simulink model "MSDR_v1"  (R2018a)
settings: Solver=ode23tb  StartTime=0.0  StopTime=50000  RelTol=1e-3
values from neighbouring files (symbols this model uses):
  a_f = -3.22E-5    (= -3.22e-05)    [MSDR_parameters.m]
  a_g = +2.35E-5    (= 2.35e-05)    [MSDR_parameters.m]
  beta = [0.000223, 0.001457, 0.001307, 0.002628, 0.000766, 0.000280]    [MSDR_parameters.m]
  beta_t = sum(beta)    [MSDR_parameters.m]
  Cp_s_shx = 1549.12e-6    (= 0.00154912)    [MSDR_parameters.m]
  Cst = 10    [MSDR_parameters.m]
  dLb = 0    [MSDR_parameters.m]
  dLs = 0    [MSDR_parameters.m]
  dLsc = 0    [MSDR_parameters.m]
  gamma_I = 5.1135e-2    (= 0.051135)    [MSDR_parameters.m]
  gamma_Xe = 1.1628e-2    (= 0.011628)    [MSDR_parameters.m]
  hA_fg = [h_fg*A_fg/2, h_fg*A_fg/2]    [MSDR_parameters.m]
  hA_p_phx1 = h_p_phx*A_p_phx    [MSDR_parameters.m]
  hA_p_phx2 = h_p_phx*A_p_phx    [MSDR_parameters.m]
  hA_p_phx3 = h_p_phx*A_p_phx    [MSDR_parameters.m]
  hA_p_phx4 = h_p_phx*A_p_phx    [MSDR_parameters.m]
  hA_p_phx5 = h_p_phx*A_p_phx    [MSDR_parameters.m]
  hA_p_phx6 = h_p_phx*A_p_phx    [MSDR_parameters.m]
  hA_p_shx1 = h_p_shx*A_p_shx    [MSDR_parameters.m]
  hA_p_shx2 = h_p_shx*A_p_shx    [MSDR_parameters.m]
  hA_p_shx3 = h_p_shx*A_p_shx    [MSDR_parameters.m]
  hA_p_shx4 = h_p_shx*A_p_shx    [MSDR_parameters.m]
  hA_p_shx5 = h_p_shx*A_p_shx    [MSDR_parameters.m]
  hA_p_shx6 = h_p_shx*A_p_shx    [MSDR_parameters.m]
  hA_s_phx1 = h_s_phx*A_s_phx    [MSDR_parameters.m]
  hA_s_phx2 = h_s_phx*A_s_phx    [MSDR_parameters.m]
  hA_s_phx3 = h_s_phx*A_s_phx    [MSDR_parameters.m]
  hA_s_phx4 = h_s_phx*A_s_phx    [MSDR_parameters.m]
  hA_s_phx5 = h_s_phx*A_s_phx    [MSDR_parameters.m]
  hA_s_phx6 = h_s_phx*A_s_phx    [MSDR_parameters.m]
  hA_s_shx1 = h_s_shx*A_s_shx    [MSDR_parameters.m]
  hA_s_shx2 = h_s_shx*A_s_shx    [MSDR_parameters.m]
  hA_s_shx3 = h_s_shx*A_s_shx    [MSDR_parameters.m]
  hA_s_shx4 = h_s_shx*A_s_shx    [MSDR_parameters.m]
  hA_s_shx5 = h_s_shx*A_s_shx    [MSDR_parameters.m]
  hA_s_shx6 = h_s_shx*A_s_shx    [MSDR_parameters.m]
  I_0 = gamma_I*Sig_f_msdr*phi_0/lam_I    (= 4.38204721773e+16)    [MSDR_parameters.m]
  Ifa = [0.25, 0.25]    [MSDR_parameters.m]
  Ifb = [0.25, 0.25]    [MSDR_parameters.m]
  Ig = [0.5, 0.5]    [MSDR_parameters.m]
  J = 1e-6    (= 1e-06)    [MSDR_parameters.m]
  ka = [0.235, 0.235]    [MSDR_parameters.m]
  kb = [0.235, 0.235]    [MSDR_parameters.m]
  kc = 5    [MSDR_parameters.m]
  kga = [0.015, 0.015]    [MSDR_parameters.m]
  kgb = [0.015, 0.015]    [MSDR_parameters.m]
  L = 8.5344    [MSDR_parameters.m]
  Lam = 2.400E-04    (= 0.00024)    [MSDR_parameters.m]
  lam = [0.0124, 0.0305, 0.111, 0.301, 1.14, 3.01]    [MSDR_parameters.m]
  lam_bubl = 2.0e-2    (= 0.02)    [MSDR_parameters.m]
  lam_I = 2.875e-5    (= 2.875e-05)    [MSDR_parameters.m]
  lam_Xe = 2.0916e-5    (= 2.0916e-05)    [MSDR_parameters.m]
  m_3m = W_3*2    (= 8618.207327)    [MSDR_parameters.m]
  m_fm = W_f*2    (= 9978.96)    [MSDR_parameters.m]
  m_sb = 1717    [MSDR_parameters.m]
  mb_cpb = 2.689619410657651e+00    (= 2.68961941066)    [MSDR_parameters.m]
  mcp_fa = mfa*Cp_f    [MSDR_parameters.m]
  mcp_fb = mfb*Cp_f    [MSDR_parameters.m]
  mcp_g = mg*Cp_g    [MSDR_parameters.m]
  mcp_p_phx1 = Cp_p_phx*mp_phx1    [MSDR_parameters.m]
  mcp_p_phx2 = Cp_p_phx*mp_phx2    [MSDR_parameters.m]
  mcp_p_phx3 = Cp_p_phx*mp_phx3    [MSDR_parameters.m]
  mcp_p_phx4 = Cp_p_phx*mp_phx4    [MSDR_parameters.m]
  mcp_p_phx5 = Cp_p_phx*mp_phx5    [MSDR_parameters.m]
  mcp_p_phx6 = Cp_p_phx*mp_phx6    [MSDR_parameters.m]
  mcp_p_shx1 = Cp_p_shx*mp_shx1    [MSDR_parameters.m]
  mcp_p_shx2 = Cp_p_shx*mp_shx2    [MSDR_parameters.m]
  mcp_p_shx3 = Cp_p_shx*mp_shx3    [MSDR_parameters.m]
  mcp_p_shx4 = Cp_p_shx*mp_shx4    [MSDR_parameters.m]
  mcp_p_shx5 = Cp_p_shx*mp_shx5    [MSDR_parameters.m]
  mcp_p_shx6 = Cp_p_shx*mp_shx6    [MSDR_parameters.m]
  mcp_s_phx1 = Cp_s_phx*ms_phx1    [MSDR_parameters.m]
  mcp_s_phx2 = Cp_s_phx*ms_phx2    [MSDR_parameters.m]
  mcp_s_phx3 = Cp_s_phx*ms_phx3    [MSDR_parameters.m]
  mcp_s_phx4 = Cp_s_phx*ms_phx4    [MSDR_parameters.m]
  mcp_s_phx5 = Cp_s_phx*ms_phx5    [MSDR_parameters.m]
  mcp_s_phx6 = Cp_s_phx*ms_phx6    [MSDR_parameters.m]
  mcp_s_shx1 = Cp_s_shx*ms_shx1    [MSDR_parameters.m]
  mcp_s_shx2 = Cp_s_shx*ms_shx1    [MSDR_parameters.m]
  mcp_s_shx3 = Cp_s_shx*ms_shx1    [MSDR_parameters.m]
  mcp_s_shx4 = Cp_s_shx*ms_shx1    [MSDR_parameters.m]
  mcp_s_shx5 = Cp_s_shx*ms_shx1    [MSDR_parameters.m]
  mcp_s_shx6 = Cp_s_shx*ms_shx1    [MSDR_parameters.m]
  mcp_t_phx1 = Cp_t_phx*mt_phx1    [MSDR_parameters.m]
  mcp_t_phx2 = Cp_t_phx*mt_phx2    [MSDR_parameters.m]
  mcp_t_phx3 = Cp_t_phx*mt_phx3    [MSDR_parameters.m]
  mcp_t_phx4 = Cp_t_phx*mt_phx4    [MSDR_parameters.m]
  mcp_t_phx5 = Cp_t_phx*mt_phx5    [MSDR_parameters.m]
  mcp_t_phx6 = Cp_t_phx*mt_phx6    [MSDR_parameters.m]
  mcp_t_shx1 = Cp_t_phx*mt_shx1    [MSDR_parameters.m]
  mcp_t_shx2 = Cp_t_phx*mt_shx2    [MSDR_parameters.m]
  mcp_t_shx3 = Cp_t_phx*mt_shx3    [MSDR_parameters.m]
  mcp_t_shx4 = Cp_t_phx*mt_shx4    [MSDR_parameters.m]
  mcp_t_shx5 = Cp_t_phx*mt_shx5    [MSDR_parameters.m]
  mcp_t_shx6 = Cp_t_phx*mt_shx6    [MSDR_parameters.m]
  mfa = [mass_fn, mass_fn]    [MSDR_parameters.m]
  mfb = [mass_fn, mass_fn]    [MSDR_parameters.m]
  mp_phx1 = [494.7, 494.7, 494.7, 494.7]    [MSDR_parameters.m]
  mp_phx2 = [494.7, 494.7, 494.7, 494.7]    [MSDR_parameters.m]
  mp_phx3 = [494.7, 494.7, 494.7, 494.7]    [MSDR_parameters.m]
  mp_phx4 = [494.7, 494.7, 494.7, 494.7]    [MSDR_parameters.m]
  mp_phx5 = [494.7, 494.7, 494.7, 494.7]    [MSDR_parameters.m]
  mp_phx6 = [494.7, 494.7, 494.7, 494.7]    [MSDR_parameters.m]
  mp_phxm = (Wp_phx1 + Wp_phx2)*1    (= 1663.16)    [MSDR_parameters.m]
  mp_shx1 = [429.3, 429.3, 429.3, 429.3]    [MSDR_parameters.m]
  mp_shx2 = [429.3, 429.3, 429.3, 429.3]    [MSDR_parameters.m]
  mp_shx3 = [429.3, 429.3, 429.3, 429.3]    [MSDR_parameters.m]
  mp_shx4 = [429.3, 429.3, 429.3, 429.3]    [MSDR_parameters.m]
  mp_shx5 = [429.3, 429.3, 429.3, 429.3]    [MSDR_parameters.m]
  mp_shx6 = [429.3, 429.3, 429.3, 429.3]    [MSDR_parameters.m]
  mp_shxm = (Wp_shx1 + Wp_shx2)*1    (= 932.38)    [MSDR_parameters.m]
  ms_phx1 = [1152.5, 1152.5, 1152.5, 1152.5]    [MSDR_parameters.m]
  ms_phx2 = [1152.5, 1152.5, 1152.5, 1152.5]    [MSDR_parameters.m]
  ms_phx3 = [1152.5, 1152.5, 1152.5, 1152.5]    [MSDR_parameters.m]
  ms_phx4 = [1152.5, 1152.5, 1152.5, 1152.5]    [MSDR_parameters.m]
  ms_phx5 = [1152.5, 1152.5, 1152.5, 1152.5]    [MSDR_parameters.m]
  ms_phx6 = [1152.5, 1152.5, 1152.5, 1152.5]    [MSDR_parameters.m]
  ms_phxm = (Ws_phx1 + Ws_phx2)*1    (= 932.38)    [MSDR_parameters.m]
  ms_shx1 = [1861.5, 1861.5, 1861.5, 1861.5]    [MSDR_parameters.m]
  ms_shx2 = [1861.5, 1861.5, 1861.5, 1861.5]    [MSDR_parameters.m]
  ... (+104 more)
undefined symbols (not defined in the file or in its folder): Ak2, As, C0, Cpp, Cps, Cpsc, Cpw, Dit, Dot, hA_p_thx1, hA_p_thx2, hA_p_thx3, hA_s_thx1, hA_s_thx2, hA_s_thx3, hc0, hfg, hfw0, HFW1, hfw10, HFW2, hpw, Hr, hr0, hwb, hws, hwsc, K3, KBHP, KBLP, Lsc, mcp_p_thx1, mcp_p_thx2, mcp_p_thx3, mcp_s_thx1, mcp_s_thx2, mcp_s_thx3, mcp_t_thx1, mcp_t_thx2, mcp_t_thx3, mp_thx1, mp_thx2, mp_thx3, ms_thx1, ms_thx2, ms_thx3, Mstm, nuf, Pp2, Pp3, Pp4, Pp5
libraries: simulink x20, aerolibconvert2 x2
(part 3 of 7)

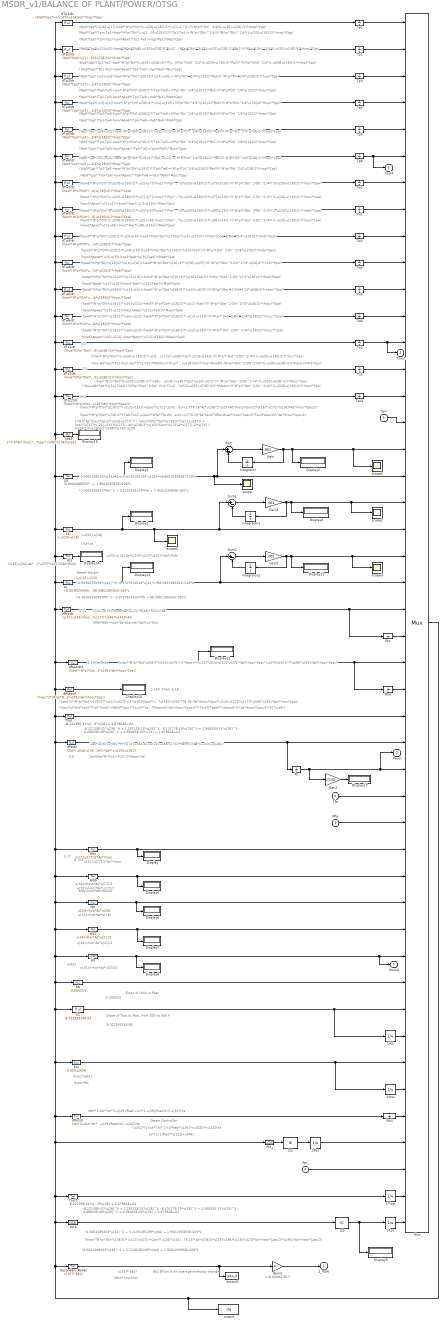
== system MSDR_v1/BALANCE OF PLANT/POWER/OTSG ==
  note: 1/(0.5*As*rhosc*Cpsc*(u[15]-u[27])) * ( hwsc*(N*pi*Dot*u[18]/2)*(u[11]-u[27]) + Cpsc*(u[31]*u[15]-u[32]*u[27]) - As*u[18]/2*(u[40]*Cpsc*(u[15]-2*u[27])-1)*u[23] ) - 0.5*As*rhosc*Cpsc*u[38]*u[18]*u[25]
  note: (u[33]-u[34]-As*u[20]*u[37]*u[25])/(As*rhob)
  note: 3.31 Ke Zhao
  note: rhosc*u[43]
  note: rhosc/Psc
  note: (Ws*(1-Cst*(kc*(1-u[29]/Pset)+kc*(1-u[29]/Pset)/ti))-u[42])/ts
  note: u[42]
  note: (0.0001589253*u[44]^2 + 0.1130185109*u[44] + 1.9561035858)/100*L
  note: (hwsc*2*(N*pi*Dot*u[18]/2)*(u[11]-u[27])+2*u[35]*Cpsc*(u[15]-u[27])-u[25]*As*u[18]*u[40]*Cpsc*(u[15]-2*u[27])+(As*u[18]*u[25]/778.16)-As*rhosc*Cpsc*(u[15]-u[27])*u[17])*u[46]*u[39]/(As*rhosc*Cpsc)
  note: u[31]-u[17]/2*As*rhosc
  note: ((hws*(N*pi*Dot*(L-u[20]-u[18])/2)*(u[8]-u[14]))-u[30]*Cps*(u[14]-u[27]))/(((N*pi*(Dot^2-Dit^2)/4*((L-u[20]-u[18])/2))*rhos)*Cps)
  note: ((hws*(N*pi*Dot*(L-u[20]-u[18])/2)*(u[7]-u[13]))-u[36]*Cps*(u[13]-u[14]))/(((N*pi*(Dot^2-Dit^2)/4*((L-u[20]-u[18])/2))*rhos)*Cps)
  note: (0.0001589253*u[44]^2 + 0.1130185109*u[44] + 1.9561035858)/100*L
  note: 882 BTU/s is an average enthalpy change
  note: u[33]*(882)
  note: Wfw*(hms-hfw)
  note: (-0.0036059099*Pth^2 - 0.3727634534*Pth + 88.5961185354)/100*L
  note: (-0.0036059099*u[44]^2 - 0.3727634534*u[44] + 88.5961185354)/100*L
  note: L-u[22]-u[18]
  note: L-Ls-Lsc
  note: (0.0001589253*Pth^2 + 0.1130185109*Pth + 1.9561035858)/100*L
  note: (0.0001589253*u[44]^2 + 0.1130185109*u[44] + 1.9561035858)/100*L
  note: 5.6
  note: u[31]+rhos*As*u[21]/2
  note: -8.22139E-31*u[26]^6 + 1.29715E-24*u[26]^5 - 8.10177E-19*u[26]^4 + 2.56855E-13*u[26]^3 - 4.48833E-08*u[26]^2 + 4.96063E-03*u[26] + 2.67964E+02
  note: Wfw-rhosc*As*dLscdt
  note: Steam Height
  note: Steam Controller
  note: (u[31]*(1-Cst*((kc*(1-(1/Pset)*u[29])+u[43])))-u[42])/ts
  note: L-u[18]-u[20]
  note: 8.02299324E-04
  note: -0.000053
  note: (u[31]-u[33]-rhosc*As*u[17])*u[46]*u[41]/(As)
  note: u[34]-rhos*As*u[21]/2
  note: -8.22139E-31*u[26]^6 + 1.29715E-24*u[26]^5 - 8.10177E-19*u[26]^4 + 2.56855E-13*u[26]^3 - 4.48833E-08*u[26]^2 + 4.96063E-03*u[26] + 2.67964E+02
  note: (hwsc*(N*pi*Dot*u[18]/2)*(u[11]-u[27])+Cpsc*(u[28]*u[15]-u[29]*u[27])+(1/778.16)*As*u[18]/2*u[25]-u[38]*u[18]*u[23]*As*rhosc*Cpsc/2)*u[38]/(As*rhosc*Cpsc/2)
  note: u[32]-rhosc*As*u[17]/2
  note: 5.17
  note: (Wfw-Wdb-rhosc*As*dLsc/dt)/(As*Lsc*Ksc)
  note: 5.13
  note: u[33]-rhob*As*u[19]
  note: 5.11
  note: 5.5
  note: 5.4
  note: ((Qs2-Wb*Cps*(u[14]-Tsat)-(((N*pi*(Dot^2-Dit^2)/4*((L-u[20]-u[18])/2))*rhos)*dHsdPs-(N*pi*(Dot^2-Dit^2)/4*((L-u[20]-u[18])/2)))*Pdots))/(((N*pi*(Dot^2-Dit^2)/4*((L-u[20]-u[18])/2))*rhos)*Cps)
  note: (Qs1-Ws*Cps*(Ts1-Ts2)-Cps*(Ts1-Ts2)*Mdots1-((N*pi*(Dot^2-Dit^2)/4*((L-u[20]-u[18])/2))*rhos)*dHsdPs-(N*pi*(Dot^2-Dit^2)/4*((L-u[20]-u[18])/2))*Pdots)/(Ms1*Cps)
  note: (hpw4*(N*pi*Dit*u[20]/2)*(u[4]-u[10])-hws4*(N*pi*Dot*u[20]/2)*(u[10]-Tsat))/(((N*pi*(Dot^2-Dit^2)/4*u[20]/2)*rhob)*Cpw)
  note: (hpw3*(N*pi*Dit*u[20]/2)*(u[3]-u[9])-hws3*(N*pi*Dot*u[20]/2)*(u[9]-Tsat))/(((N*pi*(Dot^2-Dit^2)/4*u[20]/2)*rhob)*Cpw)
  note: (hpw2*(N*pi*Dit*(L-u[20]-u[18])/2)*(u[2]-u[8])-hws2*(N*pi*Dot*(L-u[20]-u[18])/2)*(u[8]-u[14]))/(((N*pi*(Dot^2-Dit^2)/4*((L-u[20]-u[18])/2))*rhos)*Cpw)
  note: (hpw1*(N*pi*Dit*(L-u[20]-u[18])/2)*(u[1]-u[7])-hws1*(N*pi*Dot*(L-u[20]-u[18])/2)*(u[7]-u[13]))/(((N*pi*(Dot^2-Dit^2)/4*((L-u[20]-u[18])/2))*rhos)*Cpw)
  note: (Wp0*Cpp*(Tp3-Tp4)-hpw*(N*pi*Dit*u[20]/2)*(Tp4-Tw4)+(N*pi*Dit^2/4*u[20]/2)*Pp4)/(((N*pi*Dit^2/4*u[20]/2)*rhop)*Cpp)
  note: (Wp0*Cpp*(Tp2-Tp3)-hpw*(N*pi*Dit*u[20]/2)*(Tp3-Tw3)+(N*pi*Dit^2/4*u[20]/2)*Pp3)/(((N*pi*Dit^2/4*u[20]/2)*rhop)*Cpp)
  note: (Wp0*Cpp*(Tp1-Tp2)-hpw*(N*pi*Dit*(L-u[20]-u[18])/2)*(Tp2-Tw2)+(N*pi*(Dit)^2/4*(L-u[20]-u[18])/2)*Pp2)/(((N*pi*(Dit)^2/4*(L-u[20]-u[18])/2)*rhop)*Cpp)
  note: (Wp0*Cpp*(Tpin-Tp1)-hpw*(N*pi*Dit*(L-u[20]-u[18])/2)*(Tp1-Tw1)+(N*pi*(Dit)^2/4)/(((N*pi*(Dit)^2/4*(L-u[20]-u[18])/2)*rhop)*Cpp)
  note: (Wp0*Cpp*(Tp4-Tp5)-hpw*(N*pi*Dit*u[18]/2)*(Tp5-Tw5)+(N*pi*Dit^2/4*u[18]/2)*Pp5)/(((N*pi*Dit^2/4*u[18]/2)*rhop)*Cpp)
  note: (Wp0*Cpp*(Tp5-Tp6)-hpw*(N*pi*Dit*u[18]/2)*(Tp6-Tw6)+(N*pi*Dit^2/4*u[18]/2)*Pp6)/(((N*pi*Dit^2/4*u[18]/2)*rhop)*Cpp)
  note: (hpw6*(N*pi*Dit*u[18]/2)*(u[6]-u[12])-hws6*(N*pi*Dot*u[18]/2)*(u[12]-u[18]))/(((N*pi*(Dot^2-Dit^2)/4*u[18]/2)*rhosc)*Cpw)
  note: (hpw5*(N*pi*Dit*u[18]/2)*(u[5]-u[11])-hws5*(N*pi*Dot*u[18]/2)*(u[11]-Tsat))/(((N*pi*(Dot^2-Dit^2)/4*u[18]/2)*rhosc)*Cpw)
  note: (hwsc*(N*pi*Dot*u[18]/2)*(Tw6-Tsc2)+Cpsc*(Wfw*Tfw-Wsc*Tsc2)+1/778.16*As*Lsc/2*dPsc/dt-As*rhosc*Cpsc/2*Tsc2*dLsc/dt)/(As*rhosc*Cpsc/2)
  note: (Wp0*Cpp*(u[16]-u[1])-hpw*(N*pi*Dit*(L-u[20]-u[18])/2)*(u[1]-u[7]))/(((N*pi*(Dit)^2/4*(L-u[20]-u[18])/2)*rhop)*Cpp)
  note: (Wp0*Cpp*(u[1]-u[2])-hpw*(N*pi*Dit*(L-u[20]-u[18])/2)*(u[2]-u[8])+(N*pi*(Dit)^2/4*(L-u[20]-u[18])/2)*Pp2)/(((N*pi*(Dit)^2/4*(L-u[20]-u[18])/2)*rhop)*Cpp)
  note: (Wp0*Cpp*(u[2]-u[3])-hpw*(N*pi*Dit*u[20]/2)*(u[3]-u[9])+(N*pi*Dit^2/4*u[20]/2)*Pp3)/(((N*pi*Dit^2/4*u[20]/2)*rhop)*Cpp)
  note: (Wp0*Cpp*(u[3]-u[4])-hpw*(N*pi*Dit*u[20]/2)*(u[4]-u[10])+(N*pi*Dit^2/4*u[20]/2)*Pp4)/(((N*pi*Dit^2/4*u[20]/2)*rhop)*Cpp)
  note: (Wp0*Cpp*(u[5]-u[6])-hpw*(N*pi*Dit*u[18]/2)*(u[6]-u[12])+(N*pi*Dit^2/4*u[18]/2)*Pp6)/(((N*pi*Dit^2/4*u[18]/2)*rhop)*Cpp)
  note: (Wp0*Cpp*(u[4]-u[5])-hpw*(N*pi*Dit*u[18]/2)*(u[5]-u[11])+(N*pi*Dit^2/4*u[18]/2)*Pp5)/(((N*pi*Dit^2/4*u[18]/2)*rhop)*Cpp)
  note: (hpw1*(N*pi*Dit*(L-u[20]-u[18])/2)*(u[1]-u[7])-hws1*(N*pi*Dot*(L-u[20]-u[18])/2)*(u[7]-u[13]))/(((N*pi*(Dot^2-Dit^2)/4*((L-u[20]-u[18])/2))*rhos)*Cpw)
  note: (hpw2*(N*pi*Dit*(L-u[20]-u[18])/2)*(u[2]-u[8])-hws2*(N*pi*Dot*(L-u[20]-u[18])/2)*(u[8]-u[14]))/(((N*pi*(Dot^2-Dit^2)/4*((L-u[20]-u[18])/2))*rhos)*Cpw)
  note: (hpw3*(N*pi*Dit*u[20]/2)*(u[3]-u[9])-hws3*(N*pi*Dot*u[20]/2)*(u[9]-u[27]))/(((N*pi*(Dot^2-Dit^2)/4*u[20]/2)*rhob)*Cpw)
  note: (hpw4*(N*pi*Dit*u[20]/2)*(u[4]-u[10])-hws4*(N*pi*Dot*u[20]/2)*(u[10]-u[27]))/(((N*pi*(Dot^2-Dit^2)/4*u[20]/2)*rhob)*Cpw)
  note: (hpw5*(N*pi*Dit*u[18]/2)*(u[5]-u[11])-hws5*(N*pi*Dot*u[18]/2)*(u[11]-u[27]))/(((N*pi*(Dot^2-Dit^2)/4*u[18]/2)*rhosc)*Cpw)
  note: (hpw6*(N*pi*Dit*u[18]/2)*(u[6]-u[12])-hws6*(N*pi*Dot*u[18]/2)*(u[12]-u[15]))/(((N*pi*(Dot^2-Dit^2)/4*u[18]/2)*rhosc)*Cpw)
  note: (hwsc*pi*Dot*Lsc0*(Tw5-Tsat0)+Wfw0*Cpsc*(Tsc20-Tsat0)-((As*Lsc0/2)*(Ksc*Cpsc*(Tsc20-2*Tsat0)-1/778)*Pdotsc0)-(As*rhosc*Cpsc/2*((Tsc20-Tsat0)*Ldotsc0)))/(As*rhosc*Cpsc/2*(K1*Lsc0))
  note: p.152
  note: p.153, Chen, 5.18
  note: Zss*Mss*R*(Ts1+Ts2)/(2*Mstm*Vs)
  note: (Zss*(u[34]-u[36])*R*(u[13]+458.67+u[14]+458.67)/(2*Mstm))/(As*(L-u[20]-u[18]))
  note: Slope of Tsat vs Psat, from 500 to 600 F
  note: Slope of rhob vs Psat
  note: (Wp0*Cpp*(Tpin-Tp1)-hpw*Apws*(Tp1-Tw1)+Vps*Pp1)/(Mps*Cpp)
  note: (Wp0*Cpp*(Tp1-Tp2)-hpw*Apws*(Tp2-Tw2)+Vps*Pp2)/(Mps*Cpp)
  note: (Wp0*Cpp*(Tp2-Tp3)-hpw*Apwb*(Tp3-Tw3)+Vpb*Pp3)/(Mpb*Cpp)
  note: (Wp0*Cpp*(Tp3-Tp4)-hpw*Apwb*(Tp4-Tw4)+Vpb*Pp4)/(Mpb*Cpp)
  note: (Wp0*Cpp*(Tp4-Tp5)-hpw*Apwsc*(Tp5-Tw5)+Vpsc*Pp5)/(Mpsc*Cpp)
  note: (Wp0*Cpp*(Tp5-Tp6)-hpw*Apwsc*(Tp6-Tw6)+Vpsc*Pp6)/(Mpsc*Cpp)
  note: (hpw1*Apws*(u[1]-u[7])-hws1*Aws*(u[7]-u[13]))/(Mws*Cpw)
  note: (hpw2*Apws*(u[2]-u[8])-hws2*Aws*(u[8]-u[14]))/(Mws*Cpw)
  note: (hpw3*Apwb*(u[3]-u[9])-hws3*Awb*(u[9]-Tsat))/(Mwb*Cpw)
  note: (hpw4*Apwb*(u[4]-u[10])-hws4*Awb*(u[10]-Tsat))/(Mwb*Cpw)
  note: (hpw5*Apwsc*(u[5]-u[11])-hwsc*Awsc*(u[11]-Tsat))/(Mwsc*Cpw)
  note: (hpw6*Apwsc*(u[6]-u[12])-hwsc*Awsc*(u[12]-u[18]))/(Mwsc*Cpw)
  note: kc*(1-(1/Pset)*u[22])+u[46]
  note: (hwsc*(N*pi*Dot*u[18]/2)*(u[12]-u[15])+Cpsc*(u[31]*u[30]-u[32]*u[15])+1/778.16*As*u[18]/2*u[23]-As*rhosc*Cpsc/2*u[15]*u[17])/(u[18]*As*rhosc*Cpsc/2)
  note: (hwsc*(N*pi*Dot*u[18])*(u[11]-u[27])+2*Cpsc*(u[32]*u[15]-u[33]*u[27])-(As*rhosc*Cpsc*(u[27]*u[17])))*u[46]*u[39]/(As*rhosc*Cpsc)
  Wfw : Inport
  Tfw : Inport  Port=2
  Tpin : Inport  Port=3
  Pth_ : Inport  Port=4
  1/K1 : Math  Operator=reciprocal  SaturateOnIntegerOverflow=on
  1/Ksc : Math  Operator=reciprocal  SaturateOnIntegerOverflow=on
  1/Lsc : Math  Operator=reciprocal  SaturateOnIntegerOverflow=on
  1/Psc : Math  Operator=reciprocal  SaturateOnIntegerOverflow=on
  1/Tsat : Math  Operator=reciprocal  SaturateOnIntegerOverflow=on
  Display{,1..16} (17 alike) : Display
  Gain : Gain  Gain=.001
  Gain1 : Gain  Gain=.001
  Gain2 : Gain  Gain=.001
  Gain3 : Gain  Gain=1./0.000947817
  Gan2 : Gain  Gain=1/144
  IC2 : InitialCondition  Value=Psc
  IC9 : InitialCondition  Value=Lsc
  Integrator : Integrator  InitialCondition=dLsc
  Integrator1 : Integrator  InitialCondition=dLb
  Integrator2 : Integrator  InitialCondition=dLs
  K1 : Fcn  Expr=8.02299324E-04
  Kb : Fcn  Expr=-0.000053
  Ksc : Fcn  Expr=0.00042636
  Lb : Fcn  Expr=L-u[22]-u[18]
  Lb1 : Fcn  Expr=(u[33]-u[34]-As*u[20]*u[37]*u[25])/(As*rhob)
  Ls : Fcn  Expr=(-0.0036059099*u[44]^2 - 0.3727634534*u[44] + 88.5961185354)/100*L
  Lsc : Fcn  Expr=(0.0001589253*u[44]^2 + 0.1130185109*u[44] + 1.9561035858)/100*L
  Lsc1 : Fcn  Expr=u[18]
  Lsc2 : Fcn  Expr="1/(0.5*As*rhosc*Cpsc*(u[15]-u[27])) * (  hwsc*(N*pi*Dot*u[18]/2)*(u[11]-u[27])  +  Cpsc*(u[31]*u[15]-u[32]*u[27])  -  As*u[18]/2*(u[40]*Cpsc*(u[15]-2*u[27])-1)*u[23]  )  -  0.5*As*rhosc*Cpsc*u[38]*u[18]*u[25]"
  Mux : Mux  Inputs=46
      settings: DisplayOption=signals
  Ps : Integrator  InitialCondition=Ps
  Psat : Integrator  InitialCondition=Psat
  Psc : Integrator  InitialCondition=Psc
  Psc_ : Fcn  Expr=u[24]
  Secondary Power : Fcn  Expr=u[33]*(882)
  Sum : Sum  Inputs=|+-
  Sum1 : Sum  Inputs=|+-
  Sum2 : Sum  Inputs=|+-
  Tp1 : Integrator  InitialCondition=Tp1
  Tp2 : Integrator  InitialCondition=Tp2
  Tp3 : Integrator  InitialCondition=Tp3
  Tp4 : Integrator  InitialCondition=Tp4
  Tp5 : Integrator  InitialCondition=Tp5
  Tp6 : Integrator  InitialCondition=Tp6
  Ts1 : Integrator  InitialCondition=Ts1  UpperSaturationLimit=SSValue(end,13)*1.5  LowerSaturationLimit=SSValue(end,13)*0.9
  Ts2 : Integrator  InitialCondition=Ts2  UpperSaturationLimit=SSValue(end,14)*1.5  LowerSaturationLimit=SSValue(end,14)*0.9
  Tsat : Fcn  Expr=-8.22139E-31*u[26]^6 + 1.29715E-24*u[26]^5 - 8.10177E-19*u[26]^4 + 2.56855E-13*u[26]^3 - 4.48833E-08*u[26]^2 + 4.96063E-03*u[26] + 2.67964E+02
  Tsat1 : Fcn  Expr=-8.22139E-31*u[26]^6 + 1.29715E-24*u[26]^5 - 8.10177E-19*u[26]^4 + 2.56855E-13*u[26]^3 - 4.48833E-08*u[26]^2 + 4.96063E-03*u[26] + 2.67964E+02
  Tsc2 : Integrator  InitialCondition=Tsc2  UpperSaturationLimit=600  LowerSaturationLimit=515
  Tw1 : Integrator  InitialCondition=Tw1
  Tw2 : Integrator  InitialCondition=Tw2
  Tw3 : Integrator  InitialCondition=Tw3
  Tw4 : Integrator  InitialCondition=Tw4
  Tw5 : Integrator  InitialCondition=Tw5
  Tw6 : Integrator  InitialCondition=Tw6
  W12 : Fcn  Expr=u[34]-rhos*As*u[21]/2
  Wb : Fcn  Expr=u[33]-rhob*As*u[19]
  Wdb : Fcn  Expr=u[32]-rhosc*As*u[17]/2
  Ws : Fcn  Expr=u[42]
  Ws1 : Integrator  InitialCondition=Ws
  Wsc : Fcn  Expr=u[31]-u[17]/2*As*rhosc
  dPs/dt : Fcn  Expr=(Zss*(u[34]-u[36])*R*(u[13]+458.67+u[14]+458.67)/(2*Mstm))/(As*(L-u[20]-u[18]))
  dPsat/dt : Fcn  Expr=(hwsc*2*(N*pi*Dot*u[18]/2)*(u[11]-u[27])+2*u[35]*Cpsc*(u[15]-u[27])-u[25]*As*u[18]*u[40]*Cpsc*(u[15]-2*u[27])+(As*u[18]*u[25]/778.16)-As*rhosc*Cpsc*(u[15]-u[27])*u[17])*u[46]*u[39]/(As*rhosc*Cpsc)
  dPsat/dt2 : Fcn  Expr=(hwsc*(N*pi*Dot*u[18])*(u[11]-u[27])+2*Cpsc*(u[32]*u[15]-u[33]*u[27])-(As*rhosc*Cpsc*(u[27]*u[17])))*u[46]*u[39]/(As*rhosc*Cpsc)
  dPsc/dt : Fcn  Expr=(u[31]-u[33]-rhosc*As*u[17])*u[46]*u[41]/(As)
  dTp1/dt : Fcn  Expr=(Wp0*Cpp*(u[16]-u[1])-hpw*(N*pi*Dit*(L-u[20]-u[18])/2)*(u[1]-u[7]))/(((N*pi*(Dit)^2/4*(L-u[20]-u[18])/2)*rhop)*Cpp)
  dTp2/dt : Fcn  Expr=(Wp0*Cpp*(u[1]-u[2])-hpw*(N*pi*Dit*(L-u[20]-u[18])/2)*(u[2]-u[8])+(N*pi*(Dit)^2/4*(L-u[20]-u[18])/2)*Pp2)/(((N*pi*(Dit)^2/4*(L-u[20]-u[18])/2)*rhop)*Cpp)
  dTp3/dt : Fcn  Expr=(Wp0*Cpp*(u[2]-u[3])-hpw*(N*pi*Dit*u[20]/2)*(u[3]-u[9])+(N*pi*Dit^2/4*u[20]/2)*Pp3)/(((N*pi*Dit^2/4*u[20]/2)*rhop)*Cpp)
  dTp4/dt : Fcn  Expr=(Wp0*Cpp*(u[3]-u[4])-hpw*(N*pi*Dit*u[20]/2)*(u[4]-u[10])+(N*pi*Dit^2/4*u[20]/2)*Pp4)/(((N*pi*Dit^2/4*u[20]/2)*rhop)*Cpp)
  dTp5/dt : Fcn  Expr=(Wp0*Cpp*(u[4]-u[5])-hpw*(N*pi*Dit*u[18]/2)*(u[5]-u[11])+(N*pi*Dit^2/4*u[18]/2)*Pp5)/(((N*pi*Dit^2/4*u[18]/2)*rhop)*Cpp)
  dTp6/dt : Fcn  Expr=(Wp0*Cpp*(u[5]-u[6])-hpw*(N*pi*Dit*u[18]/2)*(u[6]-u[12])+(N*pi*Dit^2/4*u[18]/2)*Pp6)/(((N*pi*Dit^2/4*u[18]/2)*rhop)*Cpp)
  dTs1/dt : Fcn  Expr=((hws*(N*pi*Dot*(L-u[20]-u[18])/2)*(u[7]-u[13]))-u[36]*Cps*(u[13]-u[14]))/(((N*pi*(Dot^2-Dit^2)/4*((L-u[20]-u[18])/2))*rhos)*Cps)
  dTs2/dt : Fcn  Expr=((hws*(N*pi*Dot*(L-u[20]-u[18])/2)*(u[8]-u[14]))-u[34]*Cps*(u[14]-u[27]))/(((N*pi*(Dot^2-Dit^2)/4*((L-u[20]-u[18])/2))*rhos)*Cps)
  dTsc2/dt : Fcn  Expr=(hwsc*(N*pi*Dot*u[18]/2)*(u[12]-u[15])+Cpsc*(u[31]*u[30]-u[32]*u[15])+1/778.16*As*u[18]/2*u[23]-As*rhosc*Cpsc/2*u[15]*u[17])/(u[18]*As*rhosc*Cpsc/2)
  dTw1/dt : Fcn  Expr=(hpw*(N*pi*Dit*(L-u[20]-u[18])/2)*(u[1]-u[7])-hws*(N*pi*Dot*(L-u[20]-u[18])/2)*(u[7]-u[13]))/(((N*pi*(Dot^2-Dit^2)/4*((L-u[20]-u[18])/2))*rhos)*Cpw)
  dTw2/dt : Fcn  Expr=(hpw*(N*pi*Dit*(L-u[20]-u[18])/2)*(u[2]-u[8])-hws*(N*pi*Dot*(L-u[20]-u[18])/2)*(u[8]-u[14]))/(((N*pi*(Dot^2-Dit^2)/4*((L-u[20]-u[18])/2))*rhos)*Cpw)
  dTw3/dt : Fcn  Expr=(hpw*(N*pi*Dit*u[20]/2)*(u[3]-u[9])-hwb*(N*pi*Dot*u[20]/2)*(u[9]-u[27]))/(((N*pi*(Dot^2-Dit^2)/4*u[20]/2)*rhob)*Cpw)
  dTw4/dt : Fcn  Expr=(hpw*(N*pi*Dit*u[20]/2)*(u[4]-u[10])-hwb*(N*pi*Dot*u[20]/2)*(u[10]-u[27]))/(((N*pi*(Dot^2-Dit^2)/4*u[20]/2)*rhob)*Cpw)
  dTw5/dt : Fcn  Expr=(hpw*(N*pi*Dit*u[18]/2)*(u[5]-u[11])-hwsc*(N*pi*Dot*u[18]/2)*(u[11]-u[27]))/(((N*pi*(Dot^2-Dit^2)/4*u[18]/2)*rhosc)*Cpw)
  dTw6/dt : Fcn  Expr=(hpw*(N*pi*Dit*u[18]/2)*(u[6]-u[12])-hwsc*(N*pi*Dot*u[18]/2)*(u[12]-u[15]))/(((N*pi*(Dot^2-Dit^2)/4*u[18]/2)*rhosc)*Cpw)
  dWs/dt : Fcn  Expr=(Ws*(1-Cst*(kc*(1-u[29]/Pset)+kc*(1-u[29]/Pset)/ti))-u[42])/ts
  output : ToWorkspace  VariableName=stg  SampleTime=-1
  output1 : ToWorkspace  VariableName=pow_2  SampleTime=-1
  scope{,1..3,5} (5 alike) : Scope
  Wsout : Outport
  Psout : Outport  Port=2
  Tsout : Outport  Port=3
  Tcold : Outport  Port=4
  2_POW : Outport  Port=5
  wires:
  dTp1/dt/1 -> Tp1/1
  Tp1/1 -> Mux/1
  dTp2/dt/1 -> Tp2/1
  Tp2/1 -> Mux/2
  dTp3/dt/1 -> Tp3/1
  Tp3/1 -> Mux/3
  Tp4/1 -> Mux/4
  dTp4/dt/1 -> Tp4/1
  dTw1/dt/1 -> Tw1/1
  Tw1/1 -> Mux/7
  dTw2/dt/1 -> Tw2/1
  Tw2/1 -> Mux/8
  dTw3/dt/1 -> Tw3/1
  Tw3/1 -> Mux/9
  Tw4/1 -> Mux/10
  dTw4/dt/1 -> Tw4/1
  dTs1/dt/1 -> Ts1/1
  dTs2/dt/1 -> Ts2/1
  Ts2/1 -> Mux/14
  Tp5/1 -> Mux/5
  dTp5/dt/1 -> Tp5/1
  Tp6/1 -> Tcold/1, Mux/6
  dTp6/dt/1 -> Tp6/1
  dTw5/dt/1 -> Tw5/1
  Tw5/1 -> Mux/11
  Tw6/1 -> Mux/12
  dTw6/dt/1 -> Tw6/1
  dTsc2/dt/1 -> Tsc2/1
  Tsc2/1 -> Mux/15
  Psc/1 -> Mux/24
  Psat/1 -> Mux/26
  Ps/1 -> Mux/29, Psout/1, Gan2/1
  Ts1/1 -> Tsout/1, Mux/13
  Sum/1 -> Gain/1
  Integrator/1 -> Sum/2
  Gain1/1 -> scope2/1, Mux/19, Display4/1, Integrator1/1
  Sum2/1 -> Gain2/1
  Gain2/1 -> Display12/1, scope3/1, Mux/21, Integrator2/1
  Integrator2/1 -> Sum2/2
  Sum1/1 -> Gain1/1
  Integrator1/1 -> Sum1/2
  Secondary Power/1 -> output1/1, Gain3/1
  1/K1/1 -> Mux/39
  1/Ksc/1 -> Mux/41
  Ws1/1 -> Mux/42
  Mux/1 -> output/1, Secondary Power/1, Lsc1/1, Tsat1/1, Psc_/1, dWs/dt/1, Ksc/1, K1/1, Kb/1, Ws/1, W12/1, Wb/1, Wdb/1, Wsc/1, dPs/dt/1, Tsat/1, Ls/1, Lb1/1, Lsc2/1, dTp1/dt/1, dTp2/dt/1, dTp3/dt/1, dTp4/dt/1, dTp5/dt/1, dTp6/dt/1, dTw1/dt/1, dTw2/dt/1, dTw3/dt/1, dTw4/dt/1, dTw5/dt/1, dTw6/dt/1, dTs1/dt/1, dTs2/dt/1, dTsc2/dt/1, Lsc/1, Lb/1, dPsc/dt/1, dPsat/dt2/1, dPsat/dt/1
  Wsc/1 -> Mux/32, Display/1
  Wdb/1 -> Mux/33, Display5/1
  Wb/1 -> Mux/34, Display6/1
  W12/1 -> Mux/35, Display7/1
  1/Tsat/1 -> Mux/45
  1/Lsc/1 -> Mux/46
  Gain/1 -> scope1/1, Mux/17, Display2/1, Integrator/1
  Kb/1 -> Mux/37
  Ksc/1 -> Mux/40, 1/Ksc/1
  K1/1 -> Mux/38, 1/K1/1
  dWs/dt/1 -> Ws1/1
  Pth_/1 -> Mux/44
  Lsc1/1 -> IC9/1
  Lsc/1 -> Mux/18, Sum/1, scope/1, Display3/1
  Ls/1 -> Mux/22, Sum2/1, Display13/1
  Tpin/1 -> Mux/16
  IC9/1 -> Display9/1, 1/Lsc/1
  Tsat1/1 -> 1/Tsat/1
  Tfw/1 -> Mux/30
  Wfw/1 -> Mux/31
  dPs/dt/1 -> Mux/28, Ps/1
  Tsat/1 -> Mux/27
  dPsat/dt2/1 -> Display11/1, Mux/25, Psat/1
  dPsc/dt/1 -> Mux/23, Psc/1
  Ws/1 -> Mux/36, Wsout/1, Display8/1
  Lb/1 -> Mux/20, Sum1/1, scope5/1, Display1/1
  Gan2/1 -> Display10/1
  Psc_/1 -> IC2/1
  IC2/1 -> 1/Psc/1
  1/Psc/1 -> Mux/43
  dPsat/dt/1 -> Display15/1
  Lb1/1 -> Display14/1
  Lsc2/1 -> Display16/1
  Gain3/1 -> 2_POW/1

== system MSDR_v1/BALANCE OF PLANT/POWER/Power ==
  note: 100% to 40%
  note: 40% to 80%
  note: 80% to 60%
  note: 60% to 100%
  note: 100% to 70%
  note: 70% to 100%
  note: 100% to 20%
  note: 20% to 100%
  Constant : Constant  Value=100
  Constant1 : Constant  Value=10
  Ramp1 : simulink/Sources/Ramp  slope=0.01  start=600  InitialOutput=0
  Ramp10 : simulink/Sources/Ramp  slope=-0.0005  start=900  InitialOutput=0
  Ramp11 : simulink/Sources/Ramp  slope=0.5  start=500  InitialOutput=100
  Ramp2 : simulink/Sources/Ramp  slope=-0.01  start=500  InitialOutput=100
  Ramp3 : simulink/Sources/Ramp  slope=-0.01  start=700  InitialOutput=0
  Ramp4 : simulink/Sources/Ramp  slope=800  start=800  InitialOutput=0
  Ramp5 : simulink/Sources/Ramp  slope=0.1  start=15000  InitialOutput=0
  Ramp7 : simulink/Sources/Ramp  slope=-0.1  start=10000  InitialOutput=100
  Saturation1 : Saturate  UpperLimit=inf  LowerLimit=40
  Saturation10 : Saturate  UpperLimit=inf  LowerLimit=20
  Saturation11 : Saturate  UpperLimit=80  LowerLimit=-inf
  Saturation2 : Saturate  UpperLimit=40  LowerLimit=-inf
  Saturation3 : Saturate  UpperLimit=inf  LowerLimit=-20
  Saturation4 : Saturate  UpperLimit=40  LowerLimit=-inf
  Saturation5 : Saturate  UpperLimit=inf  LowerLimit=70
  Saturation7 : Saturate  UpperLimit=30  LowerLimit=-inf
  Scope{1..2,5..6} (4 alike) : Scope
  Sum : Sum  Inputs=++++
  Sum1 : Sum
  Sum3 : Sum
  Pth : Outport
  wires:
  Saturation1/1 -> Sum/1, Scope6/1
  Ramp2/1 -> Saturation1/1
  Ramp4/1 -> Saturation4/1
  Saturation4/1 -> Sum/4
  Ramp1/1 -> Saturation2/1
  Saturation2/1 -> Sum/2
  Ramp3/1 -> Saturation3/1
  Saturation3/1 -> Sum/3
  Saturation5/1 -> Sum1/1
  Ramp7/1 -> Saturation5/1
  Ramp5/1 -> Saturation7/1
  Saturation7/1 -> Sum1/2
  Sum1/1 -> Scope2/1
  Saturation10/1 -> Sum3/1
  Ramp11/1 -> Saturation10/1
  Ramp10/1 -> Saturation11/1
  Saturation11/1 -> Sum3/2
  Sum3/1 -> Scope5/1
  Sum/1 -> Scope1/1
  Constant/1 -> Pth/1

== system MSDR_v1/HEAT EXCHANGERS/HEAT EXCHANGER LOOP 1/BOILER & REHEATER ==
  Coolant Inlet Temp : Inport
  Power Demand (Frac) : Inport  Port=2
  Fcn : Fcn  Commented=on  Expr=u[1] - u[2]*250/((Ws_shx1 + Ws_shx2)*Cp_s_shx)
  Integrator : Integrator  InitialCondition=400
  Mux : Mux  Inputs=3
      settings: DisplayOption=signals
  To Workspace : ToWorkspace  VariableName=msdr_br_mux1  SampleTime=-1
  ddt_t_b = 1/tau_b*(t_bin-t_b)-p_b/mb_cpb : Fcn  Expr=W_sb*(u(1)-u(3))/m_sb - u(2)/mb_cpb
  Coolant Exit Temp : Outport
  wires:
  Mux/1 -> ddt_t_b = 1/tau_b*(t_bin-t_b)-p_b/mb_cpb/1, To Workspace/1
  Power Demand (Frac)/1 -> Mux/2
  Coolant Inlet Temp/1 -> Mux/1
  ddt_t_b = 1/tau_b*(t_bin-t_b)-p_b/mb_cpb/1 -> Integrator/1
  Integrator/1 -> Coolant Exit Temp/1, Mux/3

== system MSDR_v1/HEAT EXCHANGERS/HEAT EXCHANGER LOOP 1/Fractional Power Demand (fractional) ==
  Add : Sum
  Constant : Constant
  Saturation : Saturate  UpperLimit=1  LowerLimit=0.2
  Saturation1 : Saturate  UpperLimit=.8  LowerLimit=0
  Slider : Subsystem  DialogController=hmiCreateDDGDialog  IsWebBlock=on  mask(MWDashboardBlock){webBlockId=20dd6961-4cd4-422a-ae50-f434dac2eac1, webBlockType=slider, ShowInLibBrowser=on, ShowInitialText=on, HMISrcModelName=MSDR_v1}
      mask prompts: webBlockId "WebBlock Id"; webBlockType "WebBlock Type"; HMISrcModelName "Source Model"
      mask help: SimulinkHMI:dialogs:SliderDialogDesc
      mask Help: helpview([docroot '/mapfiles/simulink.map'], 'hmi_slider')
      mask Display:
      | if strcmp(get_param(bdroot(gcb),'BlockDiagramType'), 'library')
      |     image([(matlabroot) '/toolbox/simulink/hmi/icons/Slider.png']);
      | end
  down 1%/min : simulink/Sources/Ramp  slope=-0.01/60  start=2500  InitialOutput=1
  up 1%/min1 : simulink/Sources/Ramp  slope=0.01/60  start=2500+3600+5000  InitialOutput=0
  Power Demand(frac) : Outport
  wires:
  down 1%/min/1 -> Saturation/1
  Saturation/1 -> Add/1
  up 1%/min1/1 -> Saturation1/1
  Saturation1/1 -> Add/2
  Constant/1 -> Power Demand(frac)/1

== system MSDR_v1/HEAT EXCHANGERS/HEAT EXCHANGER LOOP 1/PHX PRIM MIXING ==
  Tp_phx1 : Inport
  Tp_phx2 : Inport  Port=2
  p_flow_frac : Inport  Port=3
  Fcn : Fcn  Expr=u[3]*Wp_phx1/mp_phxm*(u[1]-u[4]) + u[3]*Wp_phx2/mp_phxm*(u[2]-u[4])
  Integrator : Integrator  InitialCondition=Tf_in
  Mux : Mux
  Tp_phx_mix : Outport
  wires:
  Tp_phx1/1 -> Mux/1
  Tp_phx2/1 -> Mux/2
  Mux/1 -> Fcn/1
  p_flow_frac/1 -> Mux/3
  Fcn/1 -> Integrator/1
  Integrator/1 -> Tp_phx_mix/1, Mux/4

== system MSDR_v1/HEAT EXCHANGERS/HEAT EXCHANGER LOOP 1/PHX SEC MIXING ==
  Ts_phx1 : Inport
  Ts_phx2 : Inport  Port=2
  s_flow_frac : Inport  Port=3
  Fcn : Fcn  Expr=u[3]*Ws_phx1/ms_phxm*(u[1]-u[4]) + u[3]*Ws_phx2/ms_phxm*(u[2]-u[4])
  Integrator : Integrator  InitialCondition=T0_s_phx1(4)
  Mux : Mux
  Ts_phx_mix : Outport
  wires:
  Ts_phx1/1 -> Mux/1
  Ts_phx2/1 -> Mux/2
  Mux/1 -> Fcn/1
  s_flow_frac/1 -> Mux/3
  Fcn/1 -> Integrator/1
  Integrator/1 -> Ts_phx_mix/1, Mux/4

== system MSDR_v1/HEAT EXCHANGERS/HEAT EXCHANGER LOOP 1/PHX//SHX PUMP ==
  1-D Lookup Table : Lookup_n-D  NumberOfTableDimensions=1  BreakpointsForDimension1=xdat  Table=ydat  InternalRulePriority=Speed  RndMeth=Simplest  InputSameDT=on
  Clock : Clock
  Fcn : Fcn  Expr=exp((1/tau_p)*u)
  Final convection flow rate : Constant  Value=therm_conv
  Scope : Scope
  Subtract : Sum  Inputs=-+
  Switch : Switch  Criteria=u2 > Threshold
  Transport Delay : TransportDelay  DelayTime=2000000000  InitialOutput=1
  FLOW FRACTION : Outport
  HEAT TRANSFER FRACTION : Outport  Port=2
  wires:
  Transport Delay/1 -> 1-D Lookup Table/1, Scope/1, FLOW FRACTION/1
  Clock/1 -> Fcn/1
  Switch/1 -> Transport Delay/1
  Fcn/1 -> Subtract/1, Switch/1
  Final convection flow rate/1 -> Subtract/2, Switch/3
  Subtract/1 -> Switch/2
  1-D Lookup Table/1 -> HEAT TRANSFER FRACTION/1

== system MSDR_v1/HEAT EXCHANGERS/HEAT EXCHANGER LOOP 1/PHX1 HEAT TRANSFER ==
  PRIMARY FLUID INLET TEMPERATURE : Inport
  SECONDARY FLUID INLET TEMPERATURE : Inport  Port=2
  PRIMARY FLOW FRACTION : Inport  Port=3
  PRIMARY HEAT TRANSFER FRACTION : Inport  Port=4
  SECONDARY FLOW FRACTION : Inport  Port=5
  SECONDARY HEAT TRANSFER FRACTION : Inport  Port=6
  Mux : Mux  Inputs=16
      settings: DisplayOption=signals
  To Workspace : ToWorkspace  VariableName=phx1_ht  SampleTime=-1
  Tp1_phx1 : Integrator  InitialCondition=T0_p_phx1(1)
  Tp2_phx1 : Integrator  InitialCondition=T0_p_phx1(2)
  "Tp3_phx1 " : Integrator  InitialCondition=T0_p_phx1(3)
  Tp4_phx1 : Integrator  InitialCondition=T0_p_phx1(4)
  Ts1_phx1 : Integrator  InitialCondition=T0_s_phx1(1)
  Ts2_phx1 : Integrator  InitialCondition=T0_s_phx1(2)
  Ts3_phx1 : Integrator  InitialCondition=T0_s_phx1(3)
  Ts4_phx1 : Integrator  InitialCondition=T0_s_phx1(4)
  Tt1_phx1 : Integrator  InitialCondition=T0_t_phx1(1)
  Tt2_phx1 : Integrator  InitialCondition=T0_t_phx1(2)
  d(Tp1_phx1)/dt : Fcn  Expr=(u[13]*Wp_phx1/mp_phx1(1))*(u[1] - u[3]) + (u[14]*hA_p_phx1(1)/mcp_p_phx1(1))*(u[7] - u[3])
  d(Tp2_phx1)/dt : Fcn  Expr=(u[13]*Wp_phx1/mp_phx1(2))*(u[3] - u[4]) + (u[14]*hA_p_phx1(2)/mcp_p_phx1(2))*(u[7] - u[3])
  d(Tp3_phx1)/dt : Fcn  Expr=(u[13]*Wp_phx1/mp_phx1(3))*(u[4] - u[5]) + (u[14]*hA_p_phx1(3)/mcp_p_phx1(3))*(u[8] - u[5])
  d(Tp4_phx1)/dt : Fcn  Expr=(u[13]*Wp_phx1/mp_phx1(4))*(u[5] - u[6]) + (u[14]*hA_p_phx1(4)/mcp_p_phx1(4))*(u[8] - u[5])
  d(Ts1_phx1)/dt : Fcn  Expr=(u[15]*Ws_phx1/ms_phx1(1))*(u[2] - u[9]) + (u[16]*hA_s_phx1(1)/mcp_s_phx1(1))*(u[8] - u[9])
  d(Ts2_phx1)/dt : Fcn  Expr=(u[15]*Ws_phx1/ms_phx1(2))*(u[9] - u[10]) + (u[16]*hA_s_phx1(2)/mcp_s_phx1(2))*(u[8] - u[9])
  d(Ts3_phx1)/dt : Fcn  Expr=(u[15]*Ws_phx1/ms_phx1(3))*(u[10] - u[11]) + (u[16]*hA_s_phx1(3)/mcp_s_phx1(3))*(u[7] - u[11])
  d(Ts4_phx1)/dt : Fcn  Expr=(u[15]*Ws_phx1/ms_phx1(4))*(u[11] - u[12]) + (u[16]*hA_s_phx1(4)/mcp_s_phx1(4))*(u[7] - u[11])
  d(Tt1_phx1)/dt : Fcn  Expr=(u[14]*(hA_p_phx1(1) + hA_p_phx1(2))/mcp_t_phx1(1))*(u[3] - u[7]) + (u[16]*(hA_s_phx1(1) + hA_s_phx1(2))/mcp_t_phx1(1))*(u[11] - u[7])
  d(Tt2_phx1)/dt : Fcn  Expr=(u[14]*(hA_p_phx1(3) + hA_p_phx1(4))/mcp_t_phx1(2))*(u[5] - u[8]) + (u[16]*(hA_s_phx1(3) + hA_s_phx1(4))/mcp_t_phx1(2))*(u[9] - u[8])
  PHX1 TEMPERATURES : Outport
  wires:
  Ts1_phx1/1 -> Mux/9
  Ts2_phx1/1 -> Mux/10
  d(Ts2_phx1)/dt/1 -> Ts2_phx1/1
  d(Tp4_phx1)/dt/1 -> Tp4_phx1/1
  Tt1_phx1/1 -> Mux/7
  d(Tp2_phx1)/dt/1 -> Tp2_phx1/1
  Tp4_phx1/1 -> Mux/6
  d(Tt2_phx1)/dt/1 -> Tt2_phx1/1
  SECONDARY FLUID INLET TEMPERATURE/1 -> Mux/2
  Tt2_phx1/1 -> Mux/8
  Mux/1 -> PHX1 TEMPERATURES/1, To Workspace/1, d(Ts4_phx1)/dt/1, d(Ts3_phx1)/dt/1, d(Ts1_phx1)/dt/1, d(Tt2_phx1)/dt/1, d(Tt1_phx1)/dt/1, d(Tp4_phx1)/dt/1, d(Tp3_phx1)/dt/1, d(Tp2_phx1)/dt/1, d(Tp1_phx1)/dt/1, d(Ts2_phx1)/dt/1
  d(Tp1_phx1)/dt/1 -> Tp1_phx1/1
  d(Ts4_phx1)/dt/1 -> Ts4_phx1/1
  Tp1_phx1/1 -> Mux/3
  d(Ts1_phx1)/dt/1 -> Ts1_phx1/1
  d(Ts3_phx1)/dt/1 -> Ts3_phx1/1
  Ts3_phx1/1 -> Mux/11
  Ts4_phx1/1 -> Mux/12
  "Tp3_phx1 "/1 -> Mux/5
  d(Tp3_phx1)/dt/1 -> "Tp3_phx1 "/1
  Tp2_phx1/1 -> Mux/4
  d(Tt1_phx1)/dt/1 -> Tt1_phx1/1
  PRIMARY FLUID INLET TEMPERATURE/1 -> Mux/1
  PRIMARY FLOW FRACTION/1 -> Mux/13
  PRIMARY HEAT TRANSFER FRACTION/1 -> Mux/14
  SECONDARY HEAT TRANSFER FRACTION/1 -> Mux/16
  SECONDARY FLOW FRACTION/1 -> Mux/15

== system MSDR_v1/HEAT EXCHANGERS/HEAT EXCHANGER LOOP 1/PHX1 MATERIAL TRANSPORT ==
  PHX1 TEMPERATURES : Inport
  wires:
  PHX1 TEMPERATURES/1 -> ?

== system MSDR_v1/HEAT EXCHANGERS/HEAT EXCHANGER LOOP 1/PHX2 HEAT TRANSFER ==
  PRIMARY FLUID INLET TEMPERATURE : Inport
  SECONDARY FLUID INLET TEMPERATURE : Inport  Port=2
  PRIMARY FLOW FRACTION : Inport  Port=3
  PRIMARY HEAT TRANSFER FRACTION : Inport  Port=4
  SECONDARY FLOW FRACTION : Inport  Port=5
  SECONDARY HEAT TRANSFER FRACTION : Inport  Port=6
  Mux : Mux  Inputs=16
      settings: DisplayOption=signals
  To Workspace : ToWorkspace  VariableName=phx2_ht  SampleTime=-1
  Tp1_phx2 : Integrator  InitialCondition=T0_p_phx2(1)
  Tp2_phx2 : Integrator  InitialCondition=T0_p_phx1(2)
  "Tp3_phx2 " : Integrator  InitialCondition=T0_p_phx2(3)
  Tp4_phx2 : Integrator  InitialCondition=T0_p_phx2(4)
  Ts1_phx2 : Integrator  InitialCondition=T0_s_phx2(1)
  Ts2_phx2 : Integrator  InitialCondition=T0_s_phx2(2)
  Ts3_phx2 : Integrator  InitialCondition=T0_s_phx2(3)
  Ts4_phx2 : Integrator  InitialCondition=T0_s_phx2(4)
  Tt1_phx2 : Integrator  InitialCondition=T0_t_phx2(1)
  Tt2_phx2 : Integrator  InitialCondition=T0_t_phx2(2)
  d(Tp1_phx2)/dt : Fcn  Expr=(u[13]*Wp_phx2/mp_phx2(1))*(u[1] - u[3]) + (u[14]*hA_p_phx2(1)/mcp_p_phx2(1))*(u[7] - u[3])
  d(Tp2_phx2)/dt : Fcn  Expr=(u[13]*Wp_phx2/mp_phx2(2))*(u[3] - u[4]) + (u[14]*hA_p_phx2(2)/mcp_p_phx2(2))*(u[7] - u[3])
  d(Tp3_phx2)/dt : Fcn  Expr=(u[13]*Wp_phx2/mp_phx2(3))*(u[4] - u[5]) + (u[14]*hA_p_phx2(3)/mcp_p_phx2(3))*(u[8] - u[5])
  d(Tp4_phx2)/dt : Fcn  Expr=(u[13]*Wp_phx2/mp_phx2(4))*(u[5] - u[6]) + (u[14]*hA_p_phx2(4)/mcp_p_phx2(4))*(u[8] - u[5])
  d(Ts1_phx2)/dt : Fcn  Expr=(u[15]*Ws_phx2/ms_phx2(1))*(u[2] - u[9]) + (u[16]*hA_s_phx2(1)/mcp_s_phx2(1))*(u[8] - u[9])
  d(Ts2_phx2)/dt : Fcn  Expr=(u[15]*Ws_phx2/ms_phx2(2))*(u[9] - u[10]) + (u[16]*hA_s_phx2(2)/mcp_s_phx2(2))*(u[8] - u[9])
  d(Ts3_phx2)/dt : Fcn  Expr=(u[15]*Ws_phx2/ms_phx2(3))*(u[10] - u[11]) + (u[16]*hA_s_phx2(3)/mcp_s_phx2(3))*(u[7] - u[11])
  d(Ts4_phx2)/dt : Fcn  Expr=(u[15]*Ws_phx2/ms_phx2(4))*(u[11] - u[12]) + (u[16]*hA_s_phx2(4)/mcp_s_phx2(4))*(u[7] - u[11])
  d(Tt1_phx2)/dt : Fcn  Expr=(u[14]*(hA_p_phx2(1) + hA_p_phx2(2))/mcp_t_phx2(1))*(u[3] - u[7]) + (u[16]*(hA_s_phx2(1) + hA_s_phx2(2))/mcp_t_phx2(1))*(u[11] - u[7])
  d(Tt2_phx2)/dt : Fcn  Expr=(u[14]*(hA_p_phx2(3) + hA_p_phx2(4))/mcp_t_phx2(2))*(u[5] - u[8]) + (u[16]*(hA_s_phx2(3) + hA_s_phx2(4))/mcp_t_phx2(2))*(u[9] - u[8])
  PHX2 TEMPERATURES : Outport
  wires:
  Ts1_phx2/1 -> Mux/9
  Ts2_phx2/1 -> Mux/10
  d(Ts2_phx2)/dt/1 -> Ts2_phx2/1
  d(Tp4_phx2)/dt/1 -> Tp4_phx2/1
  Tt1_phx2/1 -> Mux/7
  d(Tp2_phx2)/dt/1 -> Tp2_phx2/1
  Tp4_phx2/1 -> Mux/6
  d(Tt2_phx2)/dt/1 -> Tt2_phx2/1
  SECONDARY FLUID INLET TEMPERATURE/1 -> Mux/2
  Tt2_phx2/1 -> Mux/8
  Mux/1 -> To Workspace/1, PHX2 TEMPERATURES/1, d(Ts4_phx2)/dt/1, d(Ts3_phx2)/dt/1, d(Ts1_phx2)/dt/1, d(Tt2_phx2)/dt/1, d(Tt1_phx2)/dt/1, d(Tp4_phx2)/dt/1, d(Tp3_phx2)/dt/1, d(Tp2_phx2)/dt/1, d(Tp1_phx2)/dt/1, d(Ts2_phx2)/dt/1
  d(Tp1_phx2)/dt/1 -> Tp1_phx2/1
  d(Ts4_phx2)/dt/1 -> Ts4_phx2/1
  Tp1_phx2/1 -> Mux/3
  d(Ts1_phx2)/dt/1 -> Ts1_phx2/1
  d(Ts3_phx2)/dt/1 -> Ts3_phx2/1
  Ts3_phx2/1 -> Mux/11
  Ts4_phx2/1 -> Mux/12
  "Tp3_phx2 "/1 -> Mux/5
  d(Tp3_phx2)/dt/1 -> "Tp3_phx2 "/1
  Tp2_phx2/1 -> Mux/4
  d(Tt1_phx2)/dt/1 -> Tt1_phx2/1
  PRIMARY FLUID INLET TEMPERATURE/1 -> Mux/1
  PRIMARY FLOW FRACTION/1 -> Mux/13
  PRIMARY HEAT TRANSFER FRACTION/1 -> Mux/14
  SECONDARY FLOW FRACTION/1 -> Mux/15
  SECONDARY HEAT TRANSFER FRACTION/1 -> Mux/16

== system MSDR_v1/HEAT EXCHANGERS/HEAT EXCHANGER LOOP 1/PHX2 MATERIAL TRANSPORT ==
  PHX2 TEMPERATURES : Inport
  wires:
  PHX2 TEMPERATURES/1 -> ?

== system MSDR_v1/HEAT EXCHANGERS/HEAT EXCHANGER LOOP 1/SHX PRIM MIXING ==
  Tp_shx1 : Inport
  Tp_shx2 : Inport  Port=2
  p_flow_frac : Inport  Port=3
  Fcn : Fcn  Expr=u[3]*Wp_shx1/mp_shxm*(u[1]-u[4]) + u[3]*Wp_shx2/mp_shxm*(u[2]-u[4])
  Integrator : Integrator  InitialCondition=T0_p_shx1(4)
  Mux : Mux
  Tp_shx_mix : Outport
  wires:
  Tp_shx1/1 -> Mux/1
  Tp_shx2/1 -> Mux/2
  Mux/1 -> Fcn/1
  p_flow_frac/1 -> Mux/3
  Fcn/1 -> Integrator/1
  Integrator/1 -> Tp_shx_mix/1, Mux/4

== system MSDR_v1/HEAT EXCHANGERS/HEAT EXCHANGER LOOP 1/SHX SEC MIXING ==
  Ts_shx1 : Inport
  Ts_shx2 : Inport  Port=2
  s_flow_frac : Inport  Port=3
  Fcn : Fcn  Expr=u[3]*Ws_shx1/ms_shxm*(u[1]-u[4]) + u[3]*Ws_shx2/ms_shxm*(u[2]-u[4])
  Integrator : Integrator  InitialCondition=T0_s_shx1(4)
  Mux : Mux
  Ts_shx_mix : Outport
  wires:
  Ts_shx1/1 -> Mux/1
  Ts_shx2/1 -> Mux/2
  Mux/1 -> Fcn/1
  s_flow_frac/1 -> Mux/3
  Fcn/1 -> Integrator/1
  Integrator/1 -> Ts_shx_mix/1, Mux/4

== system MSDR_v1/HEAT EXCHANGERS/HEAT EXCHANGER LOOP 1/SHX//THX PUMP ==
  1-D Lookup Table : Lookup_n-D  NumberOfTableDimensions=1  BreakpointsForDimension1=xdat  Table=ydat  InternalRulePriority=Speed  RndMeth=Simplest  InputSameDT=on
  Clock : Clock
  Fcn : Fcn  Expr=exp((1/tau_p)*u)
  Final convection flow rate : Constant  Value=therm_conv
  Scope : Scope
  Subtract : Sum  Inputs=-+
  Switch : Switch  Criteria=u2 > Threshold
  Transport Delay : TransportDelay  DelayTime=20000000  InitialOutput=1
  FLOW FRACTION : Outport
  HEAT TRANSFER FRACTION : Outport  Port=2
  wires:
  Transport Delay/1 -> 1-D Lookup Table/1, Scope/1, FLOW FRACTION/1
  Clock/1 -> Fcn/1
  Switch/1 -> Transport Delay/1
  Fcn/1 -> Subtract/1, Switch/1
  Final convection flow rate/1 -> Subtract/2, Switch/3
  Subtract/1 -> Switch/2
  1-D Lookup Table/1 -> HEAT TRANSFER FRACTION/1

== system MSDR_v1/HEAT EXCHANGERS/HEAT EXCHANGER LOOP 1/SHX1 HEAT TRANSFER ==
  PRIMARY FLUID INLET TEMPERATURE : Inport
  SECONDARY FLUID INLET TEMPERATURE : Inport  Port=2
  PRIMARY FLOW FRACTION : Inport  Port=3
  PRIMARY HEAT TRANSFER FRACTION : Inport  Port=4
  SECONDARY FLOW FRACTION : Inport  Port=5
  SECONDARY HEAT TRANSFER FRACTION : Inport  Port=6
  Mux : Mux  Inputs=16
      settings: DisplayOption=signals
  To Workspace : ToWorkspace  VariableName=shx1_ht  SampleTime=-1
  Tp1_shx1 : Integrator  InitialCondition=T0_p_shx1(1)
  Tp2_shx1 : Integrator  InitialCondition=T0_p_shx1(2)
  "Tp3_shx1 " : Integrator  InitialCondition=T0_p_shx1(3)
  Tp4_shx1 : Integrator  InitialCondition=T0_p_shx1(4)
  Ts1_shx1 : Integrator  InitialCondition=T0_s_shx1(1)
  Ts2_shx1 : Integrator  InitialCondition=T0_s_shx1(2)
  Ts3_shx1 : Integrator  InitialCondition=T0_s_shx1(3)
  Ts4_shx1 : Integrator  InitialCondition=T0_s_shx1(4)
  Tt1_shx1 : Integrator  InitialCondition=T0_t_shx1(1)
  Tt2_shx1 : Integrator  InitialCondition=T0_t_shx1(2)
  d(Tp1_shx1)/dt : Fcn  Expr=(u[13]*Wp_shx1/mp_shx1(1))*(u[1] - u[3]) + (u[14]*hA_p_shx1(1)/mcp_p_shx1(1))*(u[7] - u[3])
  d(Tp2_shx1)/dt : Fcn  Expr=(u[13]*Wp_shx1/mp_shx1(2))*(u[3] - u[4]) + (u[14]*hA_p_shx1(2)/mcp_p_shx1(2))*(u[7] - u[3])
  d(Tp3_shx1)/dt : Fcn  Expr=(u[13]*Wp_shx1/mp_shx1(3))*(u[4] - u[5]) + (u[14]*hA_p_shx1(3)/mcp_p_shx1(3))*(u[8] - u[5])
  d(Tp4_shx1)/dt : Fcn  Expr=(u[13]*Wp_shx1/mp_shx1(4))*(u[5] - u[6]) + (u[14]*hA_p_shx1(4)/mcp_p_shx1(4))*(u[8] - u[5])
  d(Ts1_shx1)/dt : Fcn  Expr=(u[15]*Ws_shx1/ms_shx1(1))*(u[2] - u[9]) + (u[16]*hA_s_shx1(1)/mcp_s_shx1(1))*(u[8] - u[9])
  d(Ts2_shx1)/dt : Fcn  Expr=(u[15]*Ws_shx1/ms_shx1(2))*(u[9] - u[10]) + (u[16]*hA_s_shx1(2)/mcp_s_shx1(2))*(u[8] - u[9])
  d(Ts3_shx1)/dt : Fcn  Expr=(u[15]*Ws_shx1/ms_shx1(3))*(u[10] - u[11]) + (u[16]*hA_s_shx1(3)/mcp_s_shx1(3))*(u[7] - u[11])
  d(Ts4_shx1)/dt : Fcn  Expr=(u[15]*Ws_shx1/ms_shx1(4))*(u[11] - u[12]) + (u[16]*hA_s_shx1(4)/mcp_s_shx1(4))*(u[7] - u[11])
  d(Tt1_shx1)/dt : Fcn  Expr=(u[14]*(hA_p_shx1(1) + hA_p_shx1(2))/mcp_t_shx1(1))*(u[3] - u[7]) + (u[16]*(hA_s_shx1(1) + hA_s_shx1(2))/mcp_t_shx1(1))*(u[11] - u[7])
  d(Tt2_shx1)/dt : Fcn  Expr=(u[14]*(hA_p_shx1(3) + hA_p_shx1(4))/mcp_t_shx1(2))*(u[5] - u[8]) + (u[16]*(hA_s_shx1(3) + hA_s_shx1(4))/mcp_t_shx1(2))*(u[9] - u[8])
  SHX1 TEMPERATURES : Outport
  wires:
  Ts1_shx1/1 -> Mux/9
  Ts2_shx1/1 -> Mux/10
  d(Ts2_shx1)/dt/1 -> Ts2_shx1/1
  d(Tp4_shx1)/dt/1 -> Tp4_shx1/1
  Tt1_shx1/1 -> Mux/7
  d(Tp2_shx1)/dt/1 -> Tp2_shx1/1
  Tp4_shx1/1 -> Mux/6
  d(Tt2_shx1)/dt/1 -> Tt2_shx1/1
  SECONDARY FLUID INLET TEMPERATURE/1 -> Mux/2
  Tt2_shx1/1 -> Mux/8
  Mux/1 -> To Workspace/1, SHX1 TEMPERATURES/1, d(Ts4_shx1)/dt/1, d(Ts3_shx1)/dt/1, d(Ts2_shx1)/dt/1, d(Ts1_shx1)/dt/1, d(Tt2_shx1)/dt/1, d(Tt1_shx1)/dt/1, d(Tp4_shx1)/dt/1, d(Tp3_shx1)/dt/1, d(Tp2_shx1)/dt/1, d(Tp1_shx1)/dt/1
  d(Tp1_shx1)/dt/1 -> Tp1_shx1/1
  d(Ts4_shx1)/dt/1 -> Ts4_shx1/1
  Tp1_shx1/1 -> Mux/3
  d(Ts1_shx1)/dt/1 -> Ts1_shx1/1
  d(Ts3_shx1)/dt/1 -> Ts3_shx1/1
  Ts3_shx1/1 -> Mux/11
  Ts4_shx1/1 -> Mux/12
  "Tp3_shx1 "/1 -> Mux/5
  d(Tp3_shx1)/dt/1 -> "Tp3_shx1 "/1
  Tp2_shx1/1 -> Mux/4
  d(Tt1_shx1)/dt/1 -> Tt1_shx1/1
  PRIMARY FLUID INLET TEMPERATURE/1 -> Mux/1
  PRIMARY HEAT TRANSFER FRACTION/1 -> Mux/14
  SECONDARY HEAT TRANSFER FRACTION/1 -> Mux/16
  PRIMARY FLOW FRACTION/1 -> Mux/13
  SECONDARY FLOW FRACTION/1 -> Mux/15

== system MSDR_v1/HEAT EXCHANGERS/HEAT EXCHANGER LOOP 1/SHX1 MATERIAL TRANSPORT ==
  SHX1 TEMPERATURES : Inport
  wires:
  SHX1 TEMPERATURES/1 -> ?

== system MSDR_v1/HEAT EXCHANGERS/HEAT EXCHANGER LOOP 1/SHX2 HEAT TRANSFER ==
  PRIMARY FLUID INLET TEMPERATURE : Inport
  SECONDARY FLUID INLET TEMPERATURE : Inport  Port=2
  PRIMARY FLOW FRACTION : Inport  Port=3
  PRIMARY HEAT TRANSFER FRACTION : Inport  Port=4
  SECONDARY FLOW FRACTION : Inport  Port=5
  SECONDARY HEAT TRANSFER FRACTION : Inport  Port=6
  Mux : Mux  Inputs=16
      settings: DisplayOption=signals
  To Workspace : ToWorkspace  VariableName=shx2_ht  SampleTime=-1
  Tp1_shx2 : Integrator  InitialCondition=T0_p_shx2(1)
  Tp2_shx2 : Integrator  InitialCondition=T0_p_shx2(2)
  "Tp3_shx2 " : Integrator  InitialCondition=T0_p_shx2(3)
  Tp4_shx2 : Integrator  InitialCondition=T0_p_shx2(4)
  Ts1_shx2 : Integrator  InitialCondition=T0_s_shx2(1)
  Ts2_shx2 : Integrator  InitialCondition=T0_s_shx2(2)
  Ts3_shx2 : Integrator  InitialCondition=T0_s_shx2(3)
  Ts4_shx2 : Integrator  InitialCondition=T0_s_shx2(4)
  Tt1_shx2 : Integrator  InitialCondition=T0_t_shx2(1)
  Tt2_shx2 : Integrator  InitialCondition=T0_t_shx2(2)
  d(Tp1_shx2)/dt : Fcn  Expr=(u[13]*Wp_shx2/mp_shx2(1))*(u[1] - u[3]) + (u[14]*hA_p_shx2(1)/mcp_p_shx2(1))*(u[7] - u[3])
  d(Tp2_shx2)/dt : Fcn  Expr=(u[13]*Wp_shx2/mp_shx2(2))*(u[3] - u[4]) + (u[14]*hA_p_shx2(2)/mcp_p_shx2(2))*(u[7] - u[3])
  d(Tp3_shx2)/dt : Fcn  Expr=(u[13]*Wp_shx2/mp_shx2(3))*(u[4] - u[5]) + (u[14]*hA_p_shx2(3)/mcp_p_shx2(3))*(u[8] - u[5])
  d(Tp4_shx2)/dt : Fcn  Expr=(u[13]*Wp_shx2/mp_shx2(4))*(u[5] - u[6]) + (u[14]*hA_p_shx2(4)/mcp_p_shx2(4))*(u[8] - u[5])
  d(Ts1_shx2)/dt : Fcn  Expr=(u[15]*Ws_shx2/ms_shx2(1))*(u[2] - u[9]) + (u[16]*hA_s_shx2(1)/mcp_s_shx2(1))*(u[8] - u[9])
  d(Ts2_shx2)/dt : Fcn  Expr=(u[15]*Ws_shx2/ms_shx2(2))*(u[9] - u[10]) + (u[16]*hA_s_shx2(2)/mcp_s_shx2(2))*(u[8] - u[9])
  d(Ts3_shx2)/dt : Fcn  Expr=(u[15]*Ws_shx2/ms_shx2(3))*(u[10] - u[11]) + (u[16]*hA_s_shx2(3)/mcp_s_shx2(3))*(u[7] - u[11])
  d(Ts4_shx2)/dt : Fcn  Expr=(u[15]*Ws_shx2/ms_shx2(4))*(u[11] - u[12]) + (u[16]*hA_s_shx2(4)/mcp_s_shx2(4))*(u[7] - u[11])
  d(Tt1_shx2)/dt : Fcn  Expr=(u[14]*(hA_p_shx2(1) + hA_p_shx2(2))/mcp_t_shx2(1))*(u[3] - u[7]) + (u[16]*(hA_s_shx2(1) + hA_s_shx2(2))/mcp_t_shx2(1))*(u[11] - u[7])
  d(Tt2_shx2)/dt : Fcn  Expr=(u[14]*(hA_p_shx2(3) + hA_p_shx2(4))/mcp_t_shx2(2))*(u[5] - u[8]) + (u[16]*(hA_s_shx2(3) + hA_s_shx2(4))/mcp_t_shx2(2))*(u[9] - u[8])
  SHX2 TEMPERATURES : Outport
  wires:
  Ts1_shx2/1 -> Mux/9
  Ts2_shx2/1 -> Mux/10
  d(Ts2_shx2)/dt/1 -> Ts2_shx2/1
  d(Tp4_shx2)/dt/1 -> Tp4_shx2/1
  Tt1_shx2/1 -> Mux/7
  d(Tp2_shx2)/dt/1 -> Tp2_shx2/1
  Tp4_shx2/1 -> Mux/6
  d(Tt2_shx2)/dt/1 -> Tt2_shx2/1
  SECONDARY FLUID INLET TEMPERATURE/1 -> Mux/2
  Tt2_shx2/1 -> Mux/8
  Mux/1 -> To Workspace/1, SHX2 TEMPERATURES/1, d(Ts4_shx2)/dt/1, d(Ts3_shx2)/dt/1, d(Ts2_shx2)/dt/1, d(Ts1_shx2)/dt/1, d(Tt2_shx2)/dt/1, d(Tt1_shx2)/dt/1, d(Tp4_shx2)/dt/1, d(Tp3_shx2)/dt/1, d(Tp2_shx2)/dt/1, d(Tp1_shx2)/dt/1
  d(Tp1_shx2)/dt/1 -> Tp1_shx2/1
  d(Ts4_shx2)/dt/1 -> Ts4_shx2/1
  Tp1_shx2/1 -> Mux/3
  d(Ts1_shx2)/dt/1 -> Ts1_shx2/1
  d(Ts3_shx2)/dt/1 -> Ts3_shx2/1
  Ts3_shx2/1 -> Mux/11
  Ts4_shx2/1 -> Mux/12
  "Tp3_shx2 "/1 -> Mux/5
  d(Tp3_shx2)/dt/1 -> "Tp3_shx2 "/1
  Tp2_shx2/1 -> Mux/4
  d(Tt1_shx2)/dt/1 -> Tt1_shx2/1
  PRIMARY FLUID INLET TEMPERATURE/1 -> Mux/1
  PRIMARY HEAT TRANSFER FRACTION/1 -> Mux/14
  SECONDARY FLOW FRACTION/1 -> Mux/15
  SECONDARY HEAT TRANSFER FRACTION/1 -> Mux/16
  PRIMARY FLOW FRACTION/1 -> Mux/13

== system MSDR_v1/HEAT EXCHANGERS/HEAT EXCHANGER LOOP 1/SHX2 MATERIAL TRANSPORT ==
  SHX2 TEMPERATURES : Inport
  wires:
  SHX2 TEMPERATURES/1 -> ?

== system MSDR_v1/HEAT EXCHANGERS/HEAT EXCHANGER LOOP 2/BOILER & REHEATER ==
  Coolant Inlet Temp : Inport
  Power Demand (Frac) : Inport  Port=2
  Fcn : Fcn  Commented=on  Expr=u[1] - u[2]*250/((Ws_shx1 + Ws_shx2)*Cp_s_shx)
  Integrator : Integrator  InitialCondition=400
  Mux : Mux  Inputs=3
      settings: DisplayOption=signals
  To Workspace : ToWorkspace  VariableName=msdr_br_mux2  SampleTime=-1
  ddt_t_b = 1/tau_b*(t_bin-t_b)-p_b/mb_cpb : Fcn  Expr=W_sb*(u(1)-u(3))/m_sb - u(2)/mb_cpb
  Coolant Exit Temp : Outport
  wires:
  Integrator/1 -> Coolant Exit Temp/1, Mux/3
  Mux/1 -> ddt_t_b = 1/tau_b*(t_bin-t_b)-p_b/mb_cpb/1, To Workspace/1
  Power Demand (Frac)/1 -> Mux/2
  Coolant Inlet Temp/1 -> Mux/1
  ddt_t_b = 1/tau_b*(t_bin-t_b)-p_b/mb_cpb/1 -> Integrator/1

== system MSDR_v1/HEAT EXCHANGERS/HEAT EXCHANGER LOOP 2/Fractional Power Demand (fractional) ==
  Add : Sum
  Constant : Constant
  Saturation : Saturate  UpperLimit=1  LowerLimit=0.2
  Saturation1 : Saturate  UpperLimit=.8  LowerLimit=0
  Slider : Subsystem  DialogController=hmiCreateDDGDialog  IsWebBlock=on  mask(MWDashboardBlock){webBlockId=d640d4ad-cb91-4634-9ac2-9a3bc57b8e2e, webBlockType=slider, ShowInLibBrowser=on, ShowInitialText=on, HMISrcModelName=[]}
      mask prompts: webBlockId "WebBlock Id"; webBlockType "WebBlock Type"; HMISrcModelName "Source Model"
      mask help: SimulinkHMI:dialogs:SliderDialogDesc
      mask Help: helpview([docroot '/mapfiles/simulink.map'], 'hmi_slider')
      mask Display:
      | if strcmp(get_param(bdroot(gcb),'BlockDiagramType'), 'library')
      |     image([(matlabroot) '/toolbox/simulink/hmi/icons/Slider.png']);
      | end
  down 1%/min : simulink/Sources/Ramp  slope=-0.01/60  start=2500  InitialOutput=1
  up 1%/min1 : simulink/Sources/Ramp  slope=0.01/60  start=2500+3600+5000  InitialOutput=0
  Power Demand(frac) : Outport
  wires:
  down 1%/min/1 -> Saturation/1
  Saturation/1 -> Add/1
  up 1%/min1/1 -> Saturation1/1
  Saturation1/1 -> Add/2
  Constant/1 -> Power Demand(frac)/1

== system MSDR_v1/HEAT EXCHANGERS/HEAT EXCHANGER LOOP 2/PHX PRIM MIXING ==
  Tp_phx3 : Inport
  Tp_phx4 : Inport  Port=2
  p_flow_frac : Inport  Port=3
  Fcn : Fcn  Expr=u[3]*Wp_phx3/mp_phxm*(u[1]-u[4]) + u[3]*Wp_phx4/mp_phxm*(u[2]-u[4])
  Integrator : Integrator  InitialCondition=Tf_in
  Mux : Mux
  Tp_phx_mix : Outport
  wires:
  Tp_phx3/1 -> Mux/1
  Tp_phx4/1 -> Mux/2
  Mux/1 -> Fcn/1
  p_flow_frac/1 -> Mux/3
  Fcn/1 -> Integrator/1
  Integrator/1 -> Tp_phx_mix/1, Mux/4

== system MSDR_v1/HEAT EXCHANGERS/HEAT EXCHANGER LOOP 2/PHX SEC MIXING ==
  Ts_phx3 : Inport
  Ts_phx4 : Inport  Port=2
  s_flow_frac : Inport  Port=3
  Fcn : Fcn  Expr=u[3]*Ws_phx3/ms_phxm*(u[1]-u[4]) + u[3]*Ws_phx4/ms_phxm*(u[2]-u[4])
  Integrator : Integrator  InitialCondition=T0_s_phx1(4)
  Mux : Mux
  Ts_phx_mix : Outport
  wires:
  Ts_phx3/1 -> Mux/1
  Ts_phx4/1 -> Mux/2
  Mux/1 -> Fcn/1
  s_flow_frac/1 -> Mux/3
  Fcn/1 -> Integrator/1
  Integrator/1 -> Ts_phx_mix/1, Mux/4

== system MSDR_v1/HEAT EXCHANGERS/HEAT EXCHANGER LOOP 2/PHX//SHX PUMP ==
  1-D Lookup Table : Lookup_n-D  NumberOfTableDimensions=1  BreakpointsForDimension1=xdat  Table=ydat  InternalRulePriority=Speed  RndMeth=Simplest  InputSameDT=on
  Clock : Clock
  Fcn : Fcn  Expr=exp((1/tau_p)*u)
  Final convection flow rate : Constant  Value=therm_conv
  Scope : Scope
  Subtract : Sum  Inputs=-+
  Switch : Switch  Criteria=u2 > Threshold
  Transport Delay : TransportDelay  DelayTime=60000000  InitialOutput=1
  FLOW FRACTION : Outport
  HEAT TRANSFER FRACTION : Outport  Port=2
  wires:
  Transport Delay/1 -> 1-D Lookup Table/1, Scope/1, FLOW FRACTION/1
  Clock/1 -> Fcn/1
  Switch/1 -> Transport Delay/1
  Fcn/1 -> Subtract/1, Switch/1
  Final convection flow rate/1 -> Subtract/2, Switch/3
  Subtract/1 -> Switch/2
  1-D Lookup Table/1 -> HEAT TRANSFER FRACTION/1
